simulink model "kd2bd_matched_filter_clock_extraction"  (Simulink 8.0)
settings: Solver=ode45  StartTime=0.0  StopTime=100  RelTol=1e-3
undefined symbols (not defined in the file): dfilt, fdesignblkfcn, gcbh
libraries: dsparch4 x1, commrandsrc2 x1, commsource2 x1
(part 1 of 2)
settings Model: Creator=lifes  LastModifiedBy=lifes

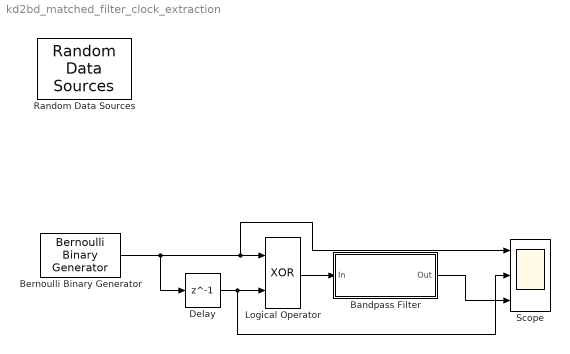
== system kd2bd_matched_filter_clock_extraction ==
  Bandpass Filter : Subsystem  DialogController=fdesignblkfcn  DialogControllerArgs=DataTag1  InitFcn=fdesignblkfcn(gcbh, {'InitFcn'});  mask(Bandpass Filter){}
      mask help: Design a bandpass filter
      settings: CopyFcn=fdesignblkfcn(gcbh, {'CopyFcn'});
      mask Help: helpview(mapfilelocation('dsp'), 'dspbandpassfilter');
      mask Display: disp('Bandpass');
  Bernoulli Binary Generator : commrandsrc2/Bernoulli Binary Generator  P=0.5  seed=61  Ts=1  frameBased=off  sampPerFrame=1  orient=off  outDataType=double
  Delay : Delay  DelayLength=1  InitialCondition=0  SampleTime=0.5
  Logical Operator : Logic  Operator=XOR  AllPortsSameDT=off  OutDataTypeStr=fixdt(1,16)  SampleTime=0.5
  Random Data Sources : commsource2/Random Data Sources
  Scope : Scope  NumInputPorts=3
      settings: YMin=-5~-5~-5  YMax=5~5~5  MaxDataPoints=100000  SampleInput=on  SampleTime=0.001
  wires:
  Bernoulli Binary Generator/1 -> Scope/1, Logical Operator/1, Delay/1
  Delay/1 -> Scope/2, Logical Operator/2
  Logical Operator/1 -> Bandpass Filter/1(In)
  Bandpass Filter/1(Out) -> Scope/3
